simulink model "MPC_rpp"  (R2024a)
settings: Solver=FixedStepAuto  StartTime=0.0  StopTime=130  FixedStep=0.05  RelTol=1e-3
PostLoadFcn:
  | on_model_load
InitFcn:
  | on_model_start
StopFcn:
  | on_simulation_done
model workspace (MAT data in the model file):
  ActiveScenario.Id = "1e727098-795b-40af-9168-30502f01196e"
  ActiveScenario.Name = "Two steps"
  ActiveScenario.Description = ""
  ActiveScenario.ConstHorizonReference = 0
  ActiveScenario.ComponentType = "scenario"
  ActiveScenario.SimulationTime = 35
  ActiveScenario.Disturbance = struct()
  ActiveScenario.Subcomponents = "Disturbance"
  ActiveScenario.SystemIc = 0
  ActiveScenario.SystemParameterOverrides = struct()
  ActiveScenario.Reference = '/home/luka/fer/csbenchlab_gym/envs/marine_otter_velocity/data/references/1e727098-795b-40af-9168-30502f01196e_ref.mat'
  ActiveScenario.DisturbanceParameterOverrides = struct()
  ActiveScenario.NumEvaluations = 1
  ActiveScenario.RandomSeed = 42
  ActiveScenario.SystemParams.payload_mass = 5.1
  ActiveScenario.SystemParams.payload_location = [0; 0; 0]
  ActiveScenario.SystemParams.current_speed = 0
  ActiveScenario.SystemParams.current_direction = 0
  ActiveScenario.SystemParams.out_gain = 1
  GlobalReference = 0
  Scenarios(1).Id = "1e727098-795b-40af-9168-30502f01196e"
  Scenarios(1).Name = "Two steps"
  Scenarios(1).Description = ""
  Scenarios(1).ConstHorizonReference = 0
  Scenarios(1).ComponentType = "scenario"
  Scenarios(1).SimulationTime = 35
  Scenarios(1).Disturbance = struct()
  Scenarios(1).Subcomponents = "Disturbance"
  Scenarios(1).SystemIc = 0
  Scenarios(1).SystemParameterOverrides = struct()
  Scenarios(1).Reference = '/home/luka/fer/csbenchlab_gym/envs/marine_otter_velocity/data/references/1e727098-795b-40af-9168-30502f01196e_ref.mat'
  Scenarios(1).DisturbanceParameterOverrides = struct()
  Scenarios(1).NumEvaluations = 1
  Scenarios(1).RandomSeed = 42
  Scenarios(2).Id = "9caafca7-6b3d-4fd5-b43b-2d0badebda60"
  Scenarios(2).Name = "Five steps perturbed"
  Scenarios(2).Description = ""
  Scenarios(2).ConstHorizonReference = 0
  Scenarios(2).ComponentType = "scenario"
  Scenarios(2).SimulationTime = 35
  Scenarios(2).Disturbance.Id = '941af73e-12e7-42cf-853d-f79bb40068e7'
  Scenarios(2).Disturbance.Name = ''
  Scenarios(2).Disturbance.Description = ''
  Scenarios(2).Disturbance.LibVersionHash = ''
  Scenarios(2).Disturbance.Lib = 'csbenchlab'
  Scenarios(2).Disturbance.LibVersion = '0.0.1'
  Scenarios(2).Disturbance.PluginType = 'dist'
  Scenarios(2).Disturbance.PluginName = 'Gauss'
  Scenarios(2).Disturbance.PluginImplementation = 'mat'
  Scenarios(2).Disturbance.ParentComponentId = '9caafca7-6b3d-4fd5-b43b-2d0badebda60'
  Scenarios(2).Disturbance.ParentComponentType = 'scenario'
  Scenarios(2).Disturbance.ComponentType = 'disturbance'
  Scenarios(2).Disturbance.DestinationPath = 'disturbances'
  Scenarios(2).Subcomponents = "Disturbance"
  Scenarios(2).SystemIc = 0
  Scenarios(2).SystemParameterOverrides = struct()
  Scenarios(2).Reference = '/home/luka/fer/csbenchlab_gym/envs/marine_otter_velocity/data/references/9caafca7-6b3d-4fd5-b43b-2d0badebda60_ref.mat'
  Scenarios(2).DisturbanceParameterOverrides = struct()
  Scenarios(2).NumEvaluations = 1000
  Scenarios(2).RandomSeed = 42
  callbacks = dictionary
  callbacks.data.Version = 1
  callbacks.data.IsKeyCombined = 1
  callbacks.data.IsValueCombined = 1
  callbacks.data.Key = ["on_start:f41ef9e4-ba34-416c-84b6-7794956a3c04"; "on_start:b11ccfb6-c361-4845-af31-0c9bdb83000b"; "on_start:0f79c310-23a7-4b0d-9134-99211e5e6d76"; "on_start:68b44e77-22b1-45f7-8742-65551543004b"; "on_start:9c6c94ce-2741-455f-a8da-be6b073916ae"; "on_start:c9039aa6-3ac2-44ce-9131-deafcda314b8"; "on_load:4a0d1010-4549-4d51-b3a5-602e7c932b45"; "on_start:4a0d1010-4549-4d51-b3a5-602e7c932b45"; "on_end:4a0d1010-4549-4d51-b3a5-602e7c932b45"]
  callbacks.data.Value{1}.external_function__ = 1
  callbacks.data.Value{1}.function = 'configure_controller_params'
  callbacks.data.Value{1}.backend = 'm'
  callbacks.data.Value{1}.kwargs = struct()
  callbacks.data.Value{2}.external_function__ = 1
  callbacks.data.Value{2}.function = 'configure_controller_params'
  callbacks.data.Value{2}.backend = 'm'
  callbacks.data.Value{2}.kwargs = struct()
  callbacks.data.Value{3}.external_function__ = 1
  callbacks.data.Value{3}.function = 'configure_controller_params'
  callbacks.data.Value{3}.backend = 'm'
  callbacks.data.Value{3}.kwargs = struct()
  callbacks.data.Value{4}.external_function__ = 1
  callbacks.data.Value{4}.function = 'configure_controller_params'
  callbacks.data.Value{4}.backend = 'm'
  callbacks.data.Value{4}.kwargs = struct()
  callbacks.data.Value{5}.external_function__ = 1
  callbacks.data.Value{5}.function = 'configure_controller_params'
  callbacks.data.Value{5}.backend = 'm'
  callbacks.data.Value{5}.kwargs = struct()
  callbacks.data.Value{6}.external_function__ = 1
  callbacks.data.Value{6}.function = 'configure_controller_params'
  callbacks.data.Value{6}.backend = 'm'
  callbacks.data.Value{6}.kwargs = struct()
  callbacks.data.Value{7} = py.function
  callbacks.data.Value{8} = py.function
  callbacks.data.Value{9} = py.function
  env_name = 'MPC_rpp'
  extrinsic = 1
  gen_blocks.systems.systems.Name = 'CS System'
  gen_blocks.systems.systems.Handle = 'MPC_rpp/CS System'
  gen_blocks.systems.systems.Path = 'MPC_rpp/CS System'
  gen_blocks.systems.systems.Disturbance = []
  gen_blocks.systems.systems.Id = "4a0d1010-4549-4d51-b3a5-602e7c932b45"
  gen_blocks.systems.systems.Components.Name = 'Otter'
  gen_blocks.systems.systems.Components.Handle = 12585.0410156
  gen_blocks.systems.systems.Components.Path = 'MPC_rpp/CS System/Otter'
  gen_blocks.systems.systems.Components.Id = "4a0d1010-4549-4d51-b3a5-602e7c932b45"
  gen_blocks.systems.systems.Components.LibPath = "marine_lib_sys/Otter"
  gen_blocks.systems.systems.SignalSubsystem = []
  gen_blocks.systems.dims.Inputs = 1
  gen_blocks.systems.dims.Outputs = 1
  gen_blocks.controllers.Name = 'CS Controller1'
  gen_blocks.controllers.Handle = 'MPC_rpp/CS Controller1'
  gen_blocks.controllers.Path = 'MPC_rpp/CS Controller1'
  gen_blocks.controllers.Id = "81fc0e6f-2384-4969-ab33-4cc0b4a88dac"
  gen_blocks.controllers.Components.Name = 'MPC'
  gen_blocks.controllers.Components.Handle = 13345.0823975
  gen_blocks.controllers.Components.Path = 'MPC_rpp/CS Controller1/MPC'
  gen_blocks.controllers.Components.Id = "81fc0e6f-2384-4969-ab33-4cc0b4a88dac"
  gen_blocks.controllers.Components.LibPath = "csbenchlab_ctl/MPC"
  gen_blocks.controllers.Components.RefExtractor.Path = 'MPC_rpp/CS Controller1/ref_extractor_1'
  gen_blocks.controllers.IoHandles.inport_y.h = 12403.0534668
  gen_blocks.controllers.IoHandles.inport_y.p.Inport = []
  gen_blocks.controllers.IoHandles.inport_y.p.Outport = 12404.0565186
  gen_blocks.controllers.IoHandles.inport_y.p.Enable = []
  gen_blocks.controllers.IoHandles.inport_y.p.Trigger = []
  gen_blocks.controllers.IoHandles.inport_y.p.State = []
  gen_blocks.controllers.IoHandles.inport_y.p.LConn = []
  gen_blocks.controllers.IoHandles.inport_y.p.RConn = []
  gen_blocks.controllers.IoHandles.inport_y.p.Ifaction = []
  gen_blocks.controllers.IoHandles.inport_y.p.Reset = []
  gen_blocks.controllers.IoHandles.inport_y.p.Event = []
  gen_blocks.controllers.IoHandles.inport_yref.h = 12401.0418701
  gen_blocks.controllers.IoHandles.inport_yref.p.Inport = []
  gen_blocks.controllers.IoHandles.inport_yref.p.Outport = 12402.0541992
  gen_blocks.controllers.IoHandles.inport_yref.p.Enable = []
  gen_blocks.controllers.IoHandles.inport_yref.p.Trigger = []
  gen_blocks.controllers.IoHandles.inport_yref.p.State = []
  gen_blocks.controllers.IoHandles.inport_yref.p.LConn = []
  gen_blocks.controllers.IoHandles.inport_yref.p.RConn = []
  gen_blocks.controllers.IoHandles.inport_yref.p.Ifaction = []
  gen_blocks.controllers.IoHandles.inport_yref.p.Reset = []
  gen_blocks.controllers.IoHandles.inport_yref.p.Event = []
  gen_blocks.controllers.IoHandles.outport_u.h = 12405.0505371
  gen_blocks.controllers.IoHandles.outport_u.p.Inport = 12406.0664062
  gen_blocks.controllers.IoHandles.outport_u.p.Outport = []
  gen_blocks.controllers.IoHandles.outport_u.p.Enable = []
  gen_blocks.controllers.IoHandles.outport_u.p.Trigger = []
  gen_blocks.controllers.IoHandles.outport_u.p.State = []
  gen_blocks.controllers.IoHandles.outport_u.p.LConn = []
  gen_blocks.controllers.IoHandles.outport_u.p.RConn = []
  gen_blocks.controllers.IoHandles.outport_u.p.Ifaction = []
  gen_blocks.controllers.IoHandles.outport_u.p.Reset = []
  gen_blocks.controllers.IoHandles.outport_u.p.Event = []
  gen_blocks.controllers.IoHandles.outport_log.h = 12407.0563965
  gen_blocks.controllers.IoHandles.outport_log.p.Inport = 12408.0462646
  gen_blocks.controllers.IoHandles.outport_log.p.Outport = []
  gen_blocks.controllers.IoHandles.outport_log.p.Enable = []
  gen_blocks.controllers.IoHandles.outport_log.p.Trigger = []
  gen_blocks.controllers.IoHandles.outport_log.p.State = []
  gen_blocks.controllers.IoHandles.outport_log.p.LConn = []
  gen_blocks.controllers.IoHandles.outport_log.p.RConn = []
  gen_blocks.controllers.IoHandles.outport_log.p.Ifaction = []
  gen_blocks.controllers.IoHandles.outport_log.p.Reset = []
  gen_blocks.controllers.IoHandles.outport_log.p.Event = []
  gen_blocks.controllers.IoHandles.in_demux.p.Inport = 31230.0020752
  gen_blocks.controllers.IoHandles.in_demux.p.Outport = 31231.0020752
  gen_blocks.controllers.IoHandles.in_demux.p.Enable = []
  gen_blocks.controllers.IoHandles.in_demux.p.Trigger = []
  gen_blocks.controllers.IoHandles.in_demux.p.State = []
  gen_blocks.controllers.IoHandles.in_demux.p.LConn = []
  gen_blocks.controllers.IoHandles.in_demux.p.RConn = []
  gen_blocks.controllers.IoHandles.in_demux.p.Ifaction = []
  gen_blocks.controllers.IoHandles.in_demux.p.Reset = []
  gen_blocks.controllers.IoHandles.in_demux.p.Event = []
  gen_blocks.controllers.IoHandles.in_demux.h = 31229.0021973
  gen_blocks.controllers.IoHandles.in_demux_ref.p.Inport = 31226.0032959
  gen_blocks.controllers.IoHandles.in_demux_ref.p.Outport = 31227.0021973
  gen_blocks.controllers.IoHandles.in_demux_ref.p.Enable = []
  gen_blocks.controllers.IoHandles.in_demux_ref.p.Trigger = []
  gen_blocks.controllers.IoHandles.in_demux_ref.p.State = []
  gen_blocks.controllers.IoHandles.in_demux_ref.p.LConn = []
  gen_blocks.controllers.IoHandles.in_demux_ref.p.RConn = []
  gen_blocks.controllers.IoHandles.in_demux_ref.p.Ifaction = []
  gen_blocks.controllers.IoHandles.in_demux_ref.p.Reset = []
  gen_blocks.controllers.IoHandles.in_demux_ref.p.Event = []
  gen_blocks.controllers.IoHandles.in_demux_ref.h = 31225.0032959
  gen_blocks.controllers.IoHandles.out_mux.p.Inport = 13313.0822754
  gen_blocks.controllers.IoHandles.out_mux.p.Outport = 13315.0822754
  gen_blocks.controllers.IoHandles.out_mux.p.Enable = []
  gen_blocks.controllers.IoHandles.out_mux.p.Trigger = []
  gen_blocks.controllers.IoHandles.out_mux.p.State = []
  gen_blocks.controllers.IoHandles.out_mux.p.LConn = []
  gen_blocks.controllers.IoHandles.out_mux.p.RConn = []
  gen_blocks.controllers.IoHandles.out_mux.p.Ifaction = []
  gen_blocks.controllers.IoHandles.out_mux.p.Reset = []
  gen_blocks.controllers.IoHandles.out_mux.p.Event = []
  gen_blocks.controllers.IoHandles.out_mux.h = 13312.0822754
  gen_blocks.controllers.IoHandles.out_mux_log.p.Inport = 13317.0822754
  gen_blocks.controllers.IoHandles.out_mux_log.p.Outport = 13319.0822754
  gen_blocks.controllers.IoHandles.out_mux_log.p.Enable = []
  gen_blocks.controllers.IoHandles.out_mux_log.p.Trigger = []
  gen_blocks.controllers.IoHandles.out_mux_log.p.State = []
  gen_blocks.controllers.IoHandles.out_mux_log.p.LConn = []
  gen_blocks.controllers.IoHandles.out_mux_log.p.RConn = []
  gen_blocks.controllers.IoHandles.out_mux_log.p.Ifaction = []
  gen_blocks.controllers.IoHandles.out_mux_log.p.Reset = []
  gen_blocks.controllers.IoHandles.out_mux_log.p.Event = []
  gen_blocks.controllers.IoHandles.out_mux_log.h = 13316.0822754
  gen_blocks.controllers.IoHandles.ref_extractors.h = 13368.0825195
  gen_blocks.controllers.IoHandles.ref_extractors.name = 'ref_extractor_1'
  gen_blocks.controllers.IoHandles.ref_extractors.p.Inport = 13371.0822754
  gen_blocks.controllers.IoHandles.ref_extractors.p.Outport = 13416.0822754
  gen_blocks.controllers.IoHandles.ref_extractors.p.Enable = []
  gen_blocks.controllers.IoHandles.ref_extractors.p.Trigger = []
  gen_blocks.controllers.IoHandles.ref_extractors.p.State = []
  gen_blocks.controllers.IoHandles.ref_extractors.p.LConn = []
  gen_blocks.controllers.IoHandles.ref_extractors.p.RConn = []
  gen_blocks.controllers.IoHandles.ref_extractors.p.Ifaction = []
  gen_blocks.controllers.IoHandles.ref_extractors.p.Reset = []
  gen_blocks.controllers.IoHandles.ref_extractors.p.Event = []
  gen_blocks.controllers.IoHandles.adapters.in_mux.h = 13425.0823975
  gen_blocks.controllers.IoHandles.adapters.in_mux.p.Inport = 13426.0823975
  gen_blocks.controllers.IoHandles.adapters.in_mux.p.Outport = 13428.0822754
  gen_blocks.controllers.IoHandles.adapters.in_mux.p.Enable = []
  gen_blocks.controllers.IoHandles.adapters.in_mux.p.Trigger = []
  gen_blocks.controllers.IoHandles.adapters.in_mux.p.State = []
  gen_blocks.controllers.IoHandles.adapters.in_mux.p.LConn = []
  gen_blocks.controllers.IoHandles.adapters.in_mux.p.RConn = []
  gen_blocks.controllers.IoHandles.adapters.in_mux.p.Ifaction = []
  gen_blocks.controllers.IoHandles.adapters.in_mux.p.Reset = []
  gen_blocks.controllers.IoHandles.adapters.in_mux.p.Event = []
  gen_blocks.controllers.IoHandles.adapters.in_mux_ref.h = 13429.0822754
  gen_blocks.controllers.IoHandles.adapters.in_mux_ref.p.Inport = 13430.0822754
  gen_blocks.controllers.IoHandles.adapters.in_mux_ref.p.Outport = 13432.0822754
  gen_blocks.controllers.IoHandles.adapters.in_mux_ref.p.Enable = []
  gen_blocks.controllers.IoHandles.adapters.in_mux_ref.p.Trigger = []
  gen_blocks.controllers.IoHandles.adapters.in_mux_ref.p.State = []
  gen_blocks.controllers.IoHandles.adapters.in_mux_ref.p.LConn = []
  gen_blocks.controllers.IoHandles.adapters.in_mux_ref.p.RConn = []
  gen_blocks.controllers.IoHandles.adapters.in_mux_ref.p.Ifaction = []
  gen_blocks.controllers.IoHandles.adapters.in_mux_ref.p.Reset = []
  gen_blocks.controllers.IoHandles.adapters.in_mux_ref.p.Event = []
  gen_blocks.controllers.IoHandles.adapters.out_demux.h = 13433.0822754
  gen_blocks.controllers.IoHandles.adapters.out_demux.p.Inport = 13434.0822754
  gen_blocks.controllers.IoHandles.adapters.out_demux.p.Outport = 13435.0822754
  gen_blocks.controllers.IoHandles.adapters.out_demux.p.Enable = []
  gen_blocks.controllers.IoHandles.adapters.out_demux.p.Trigger = []
  gen_blocks.controllers.IoHandles.adapters.out_demux.p.State = []
  gen_blocks.controllers.IoHandles.adapters.out_demux.p.LConn = []
  gen_blocks.controllers.IoHandles.adapters.out_demux.p.RConn = []
  gen_blocks.controllers.IoHandles.adapters.out_demux.p.Ifaction = []
  gen_blocks.controllers.IoHandles.adapters.out_demux.p.Reset = []
  gen_blocks.controllers.IoHandles.adapters.out_demux.p.Event = []
  gen_blocks.controllers.IoHandles.adapters.scopes.y.h = 13437.0822754
  gen_blocks.controllers.IoHandles.adapters.scopes.y.p.Inport = [13438.0822754 13441.0822754]
  gen_blocks.controllers.IoHandles.adapters.scopes.y.p.Outport = []
  gen_blocks.controllers.IoHandles.adapters.scopes.y.p.Enable = []
  gen_blocks.controllers.IoHandles.adapters.scopes.y.p.Trigger = []
  gen_blocks.controllers.IoHandles.adapters.scopes.y.p.State = []
  gen_blocks.controllers.IoHandles.adapters.scopes.y.p.LConn = []
  gen_blocks.controllers.IoHandles.adapters.scopes.y.p.RConn = []
  gen_blocks.controllers.IoHandles.adapters.scopes.y.p.Ifaction = []
  gen_blocks.controllers.IoHandles.adapters.scopes.y.p.Reset = []
  gen_blocks.controllers.IoHandles.adapters.scopes.y.p.Event = []
  gen_blocks.controllers.IoHandles.adapters.scopes.u.h = 13439.0822754
  gen_blocks.controllers.IoHandles.adapters.scopes.u.p.Inport = 13440.0822754
  gen_blocks.controllers.IoHandles.adapters.scopes.u.p.Outport = []
  gen_blocks.controllers.IoHandles.adapters.scopes.u.p.Enable = []
  gen_blocks.controllers.IoHandles.adapters.scopes.u.p.Trigger = []
  gen_blocks.controllers.IoHandles.adapters.scopes.u.p.State = []
  gen_blocks.controllers.IoHandles.adapters.scopes.u.p.LConn = []
  gen_blocks.controllers.IoHandles.adapters.scopes.u.p.RConn = []
  gen_blocks.controllers.IoHandles.adapters.scopes.u.p.Ifaction = []
  gen_blocks.controllers.IoHandles.adapters.scopes.u.p.Reset = []
  gen_blocks.controllers.IoHandles.adapters.scopes.u.p.Event = []
  gen_blocks.controllers.IoHandles.adapters.cont.h = 13345.0823975
  gen_blocks.controllers.IoHandles.adapters.cont.p.Inport = [13348.0823975 13349.0823975 13350.0823975]
  gen_blocks.controllers.IoHandles.adapters.cont.p.Outport = [13361.0822754 13362.0822754]
  gen_blocks.controllers.IoHandles.adapters.cont.p.Enable = []
  gen_blocks.controllers.IoHandles.adapters.cont.p.Trigger = []
  gen_blocks.controllers.IoHandles.adapters.cont.p.State = []
  gen_blocks.controllers.IoHandles.adapters.cont.p.LConn = []
  gen_blocks.controllers.IoHandles.adapters.cont.p.RConn = []
  gen_blocks.controllers.IoHandles.adapters.cont.p.Ifaction = []
  gen_blocks.controllers.IoHandles.adapters.cont.p.Reset = []
  gen_blocks.controllers.IoHandles.adapters.cont.p.Event = []
  gen_blocks.controllers.IoHandles.adapters.Mux.Inputs = 1
  gen_blocks.controllers.IoHandles.adapters.Mux.Outputs = 1
  gen_blocks.controllers.Estimator = []
  gen_blocks.controllers.Disturbance = []
  gen_blocks.controllers.SignalSubsystem = []
  gen_blocks.cs_blocks = {'MPC_rpp/CS Controller1'; 'MPC_rpp/CS Controller1/MPC'; 'MPC_rpp/CS System'; 'MPC_rpp/CS System/Otter'}
  gen_data_dictionary = Simulink.data.Dictionary
  id_to_params_path_map = dictionary
  id_to_params_path_map.data.Version = 1
  id_to_params_path_map.data.IsKeyCombined = 1
  id_to_params_path_map.data.IsValueCombined = 1
  id_to_params_path_map.data.Key = ["4a0d1010-4549-4d51-b3a5-602e7c932b45"; "81fc0e6f-2384-4969-ab33-4cc0b4a88dac"; "941af73e-12e7-42cf-853d-f79bb40068e7"]
  id_to_params_path_map.data.Value = ["MPC_rpp_params.sys.Otter"; "MPC_rpp_params.ctl.MPC"; "MPC_rpp_params.Subcomponents.FiveStepsPerturbed.x"]
  model_info.Metadata.Id = "e28b07d8-94b6-4791-bb8b-7f4e501fe7eb"
  model_info.Metadata.Name = "marine_otter_velocity"
  model_info.Metadata.Ts = 0.05
  model_info.Metadata.ComponentType = "metadata"
  model_info.Metadata.CoderExtrinsic = 1
  model_info.Metadata.Metadata.Authors = "Luka Mandic"
  model_info.Metadata.Metadata.Version = "0.1"
  model_info.Metadata.Metadata.License = "Apache v2"
  model_info.Metadata.Metadata.Tags = "marine,velocity"
  model_info.Metadata.Metadata.Created = ""
  model_info.Metadata.Metadata.Modified = ""
  model_info.Controllers.Id = "81fc0e6f-2384-4969-ab33-4cc0b4a88dac"
  model_info.Controllers.Name = "MPC"
  model_info.Controllers.Description = ""
  model_info.Controllers.LibVersionHash = ""
  model_info.Controllers.Lib = "csbenchlab"
  model_info.Controllers.LibVersion = "0.0.1"
  model_info.Controllers.PluginType = "ctl"
  model_info.Controllers.PluginName = "MPC"
  model_info.Controllers.IsComposable = 0
  model_info.Controllers.RefHorizon = 1
  model_info.Controllers.Mux.Inputs = 1
  model_info.Controllers.Mux.Outputs = 1
  model_info.Controllers.Subcomponents = "Subcontrollers"
  model_info.Controllers.Disturbance = struct()
  model_info.Controllers.ComponentType = "controller"
  model_info.Controllers.PluginImplementation = "slx"
  model_info.Controllers.Subcontrollers = []
  model_info.System.Id = "4a0d1010-4549-4d51-b3a5-602e7c932b45"
  model_info.System.Name = "Otter"
  model_info.System.Description = ""
  model_info.System.LibVersionHash = ""
  model_info.System.Lib = "marine_lib"
  model_info.System.LibVersion = "0.0.1"
  model_info.System.PluginType = "sys"
  model_info.System.PluginName = "Otter"
  model_info.System.Subcomponents = "Disturbance"
  model_info.System.Disturbance = struct()
  model_info.System.ComponentType = "system"
  model_info.System.PluginImplementation = "slx"
  model_info.Metrics.Id = "9c8fc09b-5b47-4f25-8326-e915b50c92f8"
  model_info.Metrics.Name = "Plot out wit reference"
  model_info.Metrics.Description = ""
  model_info.Metrics.ComponentType = "metric"
  model_info.Scenarios(1).Id = "1e727098-795b-40af-9168-30502f01196e"
  model_info.Scenarios(1).Name = "Two steps"
  model_info.Scenarios(1).Description = ""
  model_info.Scenarios(1).ConstHorizonReference = 0
  model_info.Scenarios(1).ComponentType = "scenario"
  model_info.Scenarios(1).SimulationTime = 35
  model_info.Scenarios(1).Disturbance = struct()
  model_info.Scenarios(1).Subcomponents = "Disturbance"
  model_info.Scenarios(2).Id = "9caafca7-6b3d-4fd5-b43b-2d0badebda60"
  model_info.Scenarios(2).Name = "Five steps perturbed"
  model_info.Scenarios(2).Description = ""
  model_info.Scenarios(2).ConstHorizonReference = 0
  model_info.Scenarios(2).ComponentType = "scenario"
  model_info.Scenarios(2).SimulationTime = 35
  model_info.Scenarios(2).Disturbance.Id = "941af73e-12e7-42cf-853d-f79bb40068e7"
  model_info.Scenarios(2).Disturbance.Name = ""
  model_info.Scenarios(2).Disturbance.Description = ""
  model_info.Scenarios(2).Disturbance.LibVersionHash = ""
  model_info.Scenarios(2).Disturbance.Lib = "csbenchlab"
  model_info.Scenarios(2).Disturbance.LibVersion = "0.0.1"
  model_info.Scenarios(2).Disturbance.PluginType = "dist"
  model_info.Scenarios(2).Disturbance.PluginName = "Gauss"
  model_info.Scenarios(2).Disturbance.PluginImplementation = "mat"
  model_info.Scenarios(2).Disturbance.ParentComponentId = "9caafca7-6b3d-4fd5-b43b-2d0badebda60"
  model_info.Scenarios(2).Disturbance.ParentComponentType = "scenario"
  model_info.Scenarios(2).Disturbance.ComponentType = "disturbance"
  model_info.Scenarios(2).Disturbance.DestinationPath = "disturbances"
  model_info.Scenarios(2).Disturbance.ParentComponentName = "Five steps perturbed"
  model_info.Scenarios(2).Subcomponents = "Disturbance"
  model_info.IsControlEnvironment = 0
  model_type = 'scenario'
  old_params.Subcomponents.FiveStepsPerturbed.x.mu = 0
  old_params.Subcomponents.FiveStepsPerturbed.x.sigma = 0.05
  old_params.sys.Otter.payload_mass = 5.1
  old_params.sys.Otter.payload_location = [0; 0; 0]
  old_params.sys.Otter.current_speed = 0
  old_params.sys.Otter.current_direction = 0
  old_params.sys.Otter.out_gain = 1
  old_params.ctl.MPC.mpc_path = [100 97 116 97 47 109 112 99 46 109 97 116]
  old_params.ComponentContext = dictionary
  old_params.ComponentContext.data.Version = 1
  old_params.ComponentContext.data.IsKeyCombined = 1
  old_params.ComponentContext.data.IsValueCombined = 1
  old_params.ComponentContext.data.Key = ["4a0d1010-4549-4d51-b3a5-602e7c932b45"; "81fc0e6f-2384-4969-ab33-4cc0b4a88dac"; "941af73e-12e7-42cf-853d-f79bb40068e7"]
  old_params.ComponentContext.data.Value = ["/home/luka/fer/csbenchlab_gym/envs/marine_otter_velocity/parts/systems/4a0d1010-4549-4d51-b3a5-602e7c932b45"; "/home/luka/fer/csbenchlab_gym/envs/marine_otter_velocity/parts/controllers/81fc0e6f-2384-4969-ab33-4cc0b4a88dac"; "/home/luka/fer/csbenchlab_gym/envs/marine_otter_velocity/parts/scenarios/9caafca7-6b3d-4fd5-b43b-2d0badebda60/subcomponents/disturbances/941af73e-12e7-42cf-853d-f79bb40068e7"]
  old_params.EnvPath = '/home/luka/fer/csbenchlab_gym/envs/marine_otter_velocity'
undefined symbols (not defined in the file): rpp_params
libraries: csbenchlab_ctl x1, marine_lib_sys x1, slpidlib x1, cmmi_lib x1
PostSaveFcn:
  | on_model_save
settings Model: DataDictionary=MPC_rpp_bus_types.sldd  Creator=luka  LastModifiedBy=luka

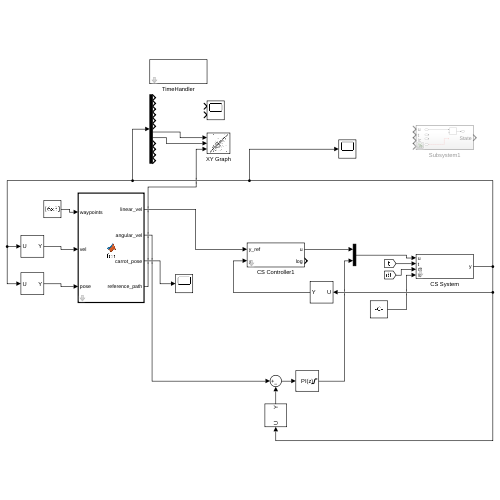
[thumbnail: Simulink's stored preview of the top-level diagram]
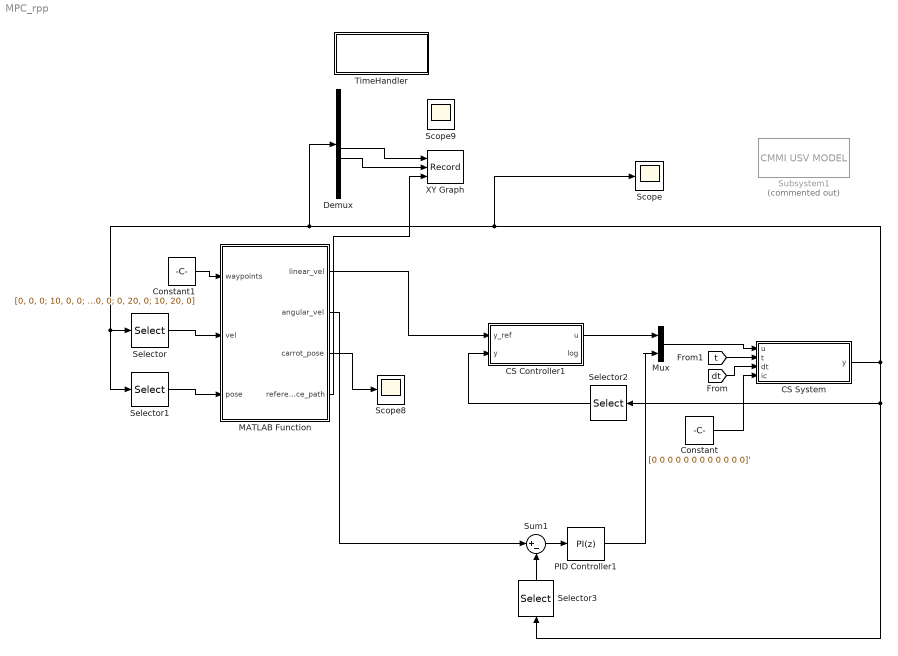
== system MPC_rpp ==
  CS Controller1 : Subsystem  Tag=__cs_template;__cs_comptype:ctl
      mask DialogControl ParameterGroupVar Prompt: Params
  CS System : Subsystem  Tag=__cs_template;__cs_comptype:sys
      mask DialogControl ParameterGroupVar Prompt: Params
  Constant : Constant  Value=[0 0 0 0 0 0 0 0 0 0 0 0]'
  Constant1 : Constant  Value=[0, 0, 0; 10, 0, 0; 10 10, 0; 0, 10, 0; 0, 20, 0; 10, 20, 0]
  Demux : Demux  Outputs=12
  MATLAB Function : MATLAB Function  TreatAsAtomicUnit=on  mask{params=rpp_params}
  Mux : Mux  Inputs=2
  PID Controller1 : slpidlib/PID Controller  Controller=PI  Form=Parallel  TimeDomain=Discrete-time  UseExternalTs=off  SampleTime=0.05  IntegratorMethod=Forward Euler  FilterMethod=Forward Euler  ControllerParametersSource=internal  P=500  I=400  UseKiTs=off  D=0.0826067692513504  UseExternalDerivativeSource=off  N=21.0121039234625  UseFilter=on  TunerSelectOption=Transfer Function Based (PID Tuner App)  InitialConditionSource=internal  InitialConditionForIntegrator=0  InitialConditionForFilter=0  DifferentiatorICPrevScaledInput=0  ExternalReset=none  TrackingMode=off  Kt=1  LimitOutput=on  SatLimitsSource=internal  UpperSaturationLimit=300  LowerSaturationLimit=-150  LinearizeAsGain=on  AntiWindupMode=clamping  Kb=1  LimitIntegrator=on  UpperIntegratorSaturationLimit=300  LowerIntegratorSaturationLimit=-150  POutMin=[]  POutMax=[]  IOutMin=[]  IOutMax=[]  DOutMin=[]  DOutMax=[]  NOutMin=[]  NOutMax=[]  SumOutMin=[]  SumOutMax=[]  SaturationOutMin=[]  SaturationOutMax=[]  PParamMin=[]  PParamMax=[]  IParamMin=[]  IParamMax=[]  DParamMin=[]  DParamMax=[]  NParamMin=[]  NParamMax=[]  KbParamMin=[]  KbParamMax=[]  KtParamMin=[]  KtParamMax=[]  KbOutMin=[]  KbOutMax=[]  KtOutMin=[]  KtOutMax=[]  IntegratorOutMin=[]  IntegratorOutMax=[]  FilterOutMin=[]  FilterOutMax=[]  SumI1OutMin=[]  SumI1OutMax=[]  SumI2OutMin=[]  SumI2OutMax=[]  SumI3OutMin=[]  SumI3OutMax=[]  SumI4OutMin=[]  SumI4OutMax=[]  SumDOutMin=[]  SumDOutMax=[]  DifferentiatorOutMin=[]  DifferentiatorOutMax=[]  FilterDiffOutCoefMin=[]  FilterDiffOutCoefMax=[]  ReciprocalOutMin=[]  ReciprocalOutMax=[]  SumDenOutMin=[]  SumDenOutMax=[]  SumNumOutMin=[]  SumNumOutMax=[]  DivideOutMin=[]  DivideOutMax=[]  UdiffTsProdOutMin=[]  UdiffTsProdOutMax=[]  NTsProdOutMin=[]  NTsProdOutMax=[]  UintegralTsProdOutMin=[]  UintegralTsProdOutMax=[]  UngainTsProdOutMin=[]  UngainTsProdOutMax=[]  ClampingZeroOutDataTypeStr=Inherit: Inherit via back propagation  ClampingZeroOutMin=[]  ClampingZeroOutMax=[]  FilterDenConstantOutDataTypeStr=Inherit: Inherit via back propagation  FilterDenConstantOutMin=[]  FilterDenConstantOutMax=[]  PCopyOutDataTypeStr=Inherit: Inherit via back propagation  PCopyOutMin=[]  PCopyOutMax=[]  NCopyOutDataTypeStr=Inherit: Inherit via back propagation  NCopyOutMin=[]  NCopyOutMax=[]  IntegratorContinuousStateAttributes=''  IntegratorStateMustResolveToSignalObject=off  IntegratorRTWStateStorageClass=Auto  FilterContinuousStateAttributes=''  FilterStateMustResolveToSignalObject=off  FilterRTWStateStorageClass=Auto  ParallelPVariant=InternalParameters  IdealPVariant=Disabled  IVariant=InternalParameters  DVariant=Disabled  IntegratorVariant=Discrete  SatVariant=Enabled  AWVariant=DiscClampingParallel  PCopyVariant=Disabled  TRVariant=Disabled  FdbkBlocksVariant=Forward  IdealPFdbkVariant=Disabled  SatFdbkVariant=Disabled  DerivativeFilterVariant=Disabled  NVariant=Disabled  NCopyVariant=Disabled_SignalSpec  FilterICVariant=Disabled  IntegratorICVariant=InternalICs  ExternalResetVariant=Disabled  TRSumVariant=Passthrough  SumFdbkVariant=Disabled  SumVariant=Sum_PI  TsampFilterVariant=InternalTs  TsampNgainVariant=Passthrough  TsampIntegralVariant=Disabled_SignalSpec  ExternalSaturationOutDataTypeStr=Inherit: Same as second input  DerivativeSourceVariant=Disabled
  Scope : Scope
  Scope8 : Scope
  Scope9 : Scope  NumInputPorts=2
  Selector : Selector  InputPortWidth=12  IndexOptions=Index vector (dialog)  Indices=[1 2 6]  OutputSizes=1
  Selector1 : Selector  InputPortWidth=12  IndexOptions=Index vector (dialog)  Indices=[7 8 12]  OutputSizes=1
  Selector2 : Selector  InputPortWidth=12  IndexOptions=Index vector (dialog)  Indices=[1]  OutputSizes=1
  Selector3 : Selector  InputPortWidth=12  IndexOptions=Index vector (dialog)  Indices=[6]  OutputSizes=1
  Subsystem1 : cmmi_lib/CMMI USV MODEL  Commented=on  SystemSampleTime=-1  VariantActivationTime=update diagram  AllowFlexibleInterface=on  Latency=0  AutoFrameSizeCalculation=off
      link override Subsystem/Saturation: UpperLimit=1  LowerLimit=-1
  Sum1 : Sum  Inputs=|+-
  TimeHandler : Subsystem
      mask DialogControl ParameterGroupVar Prompt: Params
  XY Graph : Record  FileSettingsInternal="{\"entries\":[{\"content\":{\"excelSettings\":{\"content\":{},\"type\":\"Streamout.ExcelSettings\"}},\"type\":\"Streamout.FileSettingStorage\",\"uuid\":\"\"}],\"packageUris\":[\"http:\\/\\/schema.mathworks.com\\/mf0\\/streamout_blocks\\/R2020a\"],\"version\":\"1.0\"}"  Layout=[1 1]  SignalsInternal="{\"entries\":[{\"content\":{\"signals\":[{\"content\":{\"blockPath\":[],\"dimensions\":[1],\"domain\":\"\",\"lineColor\":\"#139fff\",\"lineWidth\":2,\"port\":1,\"sid\":[\"\"],\"signalID\":1,\"signalName\":\"Demux:7\"},\"type\":\"RecordBlkView.Signal\",\"uuid\":\"\"},{\"content\":{\"blockPath\":[],\"dimensions\":[1],\"domain\":\"\",\"lineColor\":\"#ff6929\",\"lineWidth\":2,\"port\":2,\"sid\":[\"\"],\"signalID\":2,\"signalName\":\"Demux:8\"},\"type\":\"RecordBlkView.Signal\",\"uuid\":\"\"},{\"content\":{\"blockPath\":[],\"dimensions\":[501,3],\"domain\":\"\",\"hasChildren\":true,\"lineColor\":\"#b746ff\",\"lineWidth\":2,\"port\":3,\"sid\":[\"\"],\"signalID\":3,\"signalName\":\"MATLAB Function:4\"},\"type\":\"RecordBlkView.Signal\",\"uuid\":\"\"},{\"content\":{\"blockPath\":[],\"channel\":[1,1],\"dimensions\":[501,3],\"domain\":\"\",\"lineColor\":\"#64d413\",\"lineWidth\":2,\"parentID\":3,\"port\":3,\"sid\":[\"\"],\"signalID\":4,\"signalName\":\"MATLAB Function:4\"},\"type\":\"RecordBlkView.Signal\",\"uuid\":\"\"}]},\"type\":\"RecordBlkView.InputSignals\",\"uuid\":\"\"}],\"packageUris\":[\"http:\\/\\/schema.mathworks.com\\/mf0\\/streamout_blocks\\/R2020a\"],\"version\":\"1.0\"}"  VisualizationBindings="{\"xyplotplugin\":{\"info\":[{\"series\":[],\"subplotID\":1}]}}"  CompatibilityTag=XY
  wires:
  Constant1/1 -> MATLAB Function/1(waypoints)
  Selector/1 -> MATLAB Function/2(vel)
  Selector1/1 -> MATLAB Function/3(pose)
  MATLAB Function/3(carrot_pose) -> Scope8/1
  CS Controller1/1(u) -> Mux/1
  Mux/1 -> CS System/1(u)
  MATLAB Function/1(linear_vel) -> CS Controller1/1(y_ref)
  [dt] -> CS System/3(dt)
  [t] -> CS System/2(t)
  Constant/1 -> CS System/4(ic)
  Selector2/1 -> CS Controller1/2(y)
  Sum1/1 -> PID Controller1/1
  CS System/1(y) -> Selector2/1, Selector3/1, Scope/1, Selector1/1, Selector/1, Demux/1
  Selector3/1 -> Sum1/2
  MATLAB Function/2(angular_vel) -> Sum1/1
  PID Controller1/1 -> Mux/2
  MATLAB Function/4(reference_path) -> XY Graph/3
  Demux/7 -> XY Graph/1
  Demux/8 -> XY Graph/2

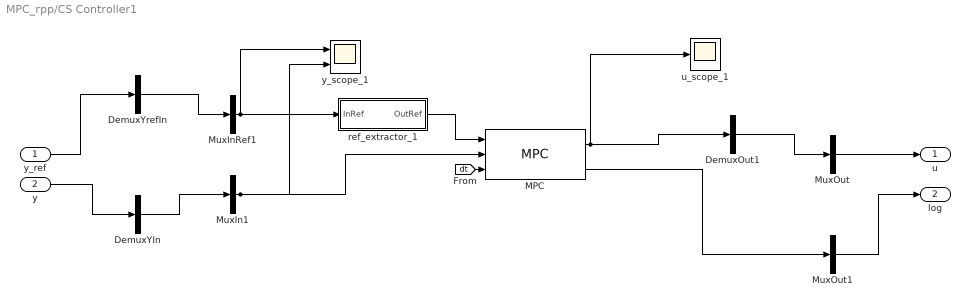
== system MPC_rpp/CS Controller1 ==
  y_ref : Inport  PortDimensions=1
  y : Inport  Port=2  PortDimensions=1
  DemuxOut1 : Demux  Outputs=1
  DemuxYIn : Demux  Outputs=1
  DemuxYrefIn : Demux  Outputs=1
  MPC : csbenchlab_ctl/MPC  Tag=__cs_slx_ctl;__cs_comptype:ctl;__cs_compimpl:slx;  mpc_path=MPC_rpp_params.ctl.MPC.mpc_path  iid__=[56 49 102 99 48 101 54 102 45 50 51 56 52 45 52 57 54 57 45 97 98 51 51 45 52 99 99 48 98 52 97 56 56 100 97 99]  pid__=[77 80 67 58 99 115 98 101 110 99 104 108 97 98]  params=MPC_rpp_params.ctl.MPC  params_struct_name=MPC_rpp_params.ctl.MPC
  MuxIn1 : Mux  Inputs=1
  MuxInRef1 : Mux  Inputs=1
  MuxOut : Mux  Inputs=1
  MuxOut1 : BusCreator  Inputs=1
  ref_extractor_1 : Subsystem
  u_scope_1 : Scope
  y_scope_1 : Scope  NumInputPorts=2
  u : Outport  PortDimensions=1
  log : Outport  Port=2
  wires:
  [dt] -> MPC/3
  y/1 -> DemuxYIn/1
  y_ref/1 -> DemuxYrefIn/1
  MuxOut/1 -> u/1
  MuxOut1/1 -> log/1
  MuxInRef1/1 -> ref_extractor_1/1(InRef), y_scope_1/1
  ref_extractor_1/1(OutRef) -> MPC/1
  MuxIn1/1 -> MPC/2, y_scope_1/2
  MPC/1 -> DemuxOut1/1, u_scope_1/1
  MPC/2 -> MuxOut1/1
  DemuxYIn/1 -> MuxIn1/1
  DemuxYrefIn/1 -> MuxInRef1/1
  DemuxOut1/1 -> MuxOut/1

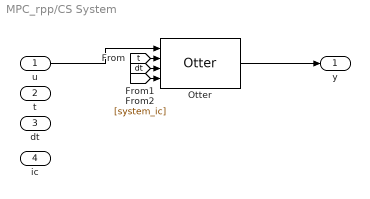
== system MPC_rpp/CS System ==
  u : Inport
  t : Inport  Port=2
  dt : Inport  Port=3
  ic : Inport  Port=4
  Otter : marine_lib_sys/Otter  Tag=system;__cs_slx_sys;__cs_comptype:sys;__cs_compimpl:slx;  payload_mass=MPC_rpp_params.sys.Otter.payload_mass  payload_location=MPC_rpp_params.sys.Otter.payload_location  current_speed=MPC_rpp_params.sys.Otter.current_speed  current_direction=MPC_rpp_params.sys.Otter.current_direction  out_gain=MPC_rpp_params.sys.Otter.out_gain  iid__=[52 97 48 100 49 48 49 48 45 52 53 52 57 45 52 100 53 49 45 98 51 97 53 45 54 48 50 101 55 99 57 51 50 98 52 53]  pid__=[79 116 116 101 114 58 109 97 114 105 110 101 95 108 105 98]  params=ActiveScenario.SystemParams  params_struct_name=MPC_rpp_params.sys.Otter
  y : Outport
  wires:
  u/1 -> Otter/1
  Otter/1 -> y/1
  [t] -> Otter/2
  [dt] -> Otter/3
  [system_ic] -> Otter/4

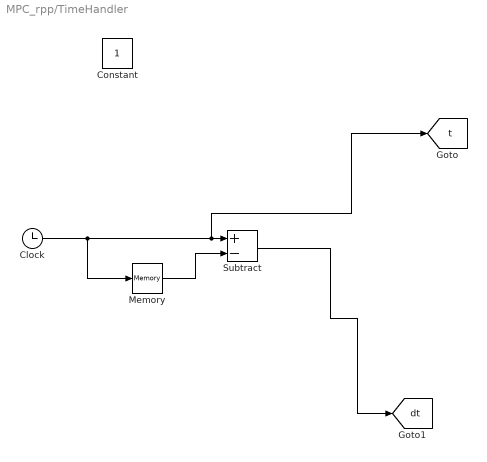
== system MPC_rpp/TimeHandler ==
  Clock : Clock
  Constant : Constant
  Memory : Memory
  Subtract : Sum  Inputs=+-
  tag scope: dt=global, t=global
  wires:
  Clock/1 -> [t], Subtract/1, Memory/1
  Memory/1 -> Subtract/2
  Subtract/1 -> [dt]

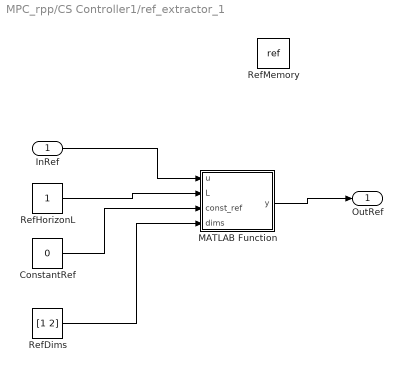
== system MPC_rpp/CS Controller1/ref_extractor_1 ==
  InRef : Inport
  ConstantRef : Constant  Value=0
  MATLAB Function : MATLAB Function  TreatAsAtomicUnit=on
  RefDims : Constant  Value=[1 2]
  RefHorizonL : Constant
  RefMemory : DataStoreMemory  DataStoreName=ref  WriteAfterWriteMsg=warning  ShowAdditionalParam=off  OutDataTypeStr=double
  OutRef : Outport
  wires:
  ConstantRef/1 -> MATLAB Function/3(const_ref)
  RefDims/1 -> MATLAB Function/4(dims)
  RefHorizonL/1 -> MATLAB Function/2(L)
  InRef/1 -> MATLAB Function/1(u)
  MATLAB Function/1(y) -> OutRef/1

== matlab function MPC_rpp/MATLAB Function ==
  settings: updateMethod=DISCRETE
  data: waypoints input; vel input; pose input; linear_vel output; params parameter; angular_vel output; carrot_pose output size=[1 3]; reference_path output
function [linear_vel, angular_vel, carrot_pose, reference_path] = fcn(waypoints, vel, pose, params)

    persistent global_path idx initial_global_path
    use_waypoints = 1;
    num_divs = 100;        
    if isempty(global_path)

        if use_waypoints
            global_path = zeros((height(waypoints)-1) * num_divs+1, 3);
            global_path(1, :) = waypoints(1, :);
            for i=1:length(waypoints)-1
                global_path(2 + (i-1)*num_divs : i*num_divs+1, :) = get_traj_between(waypoints(i, :), waypoints(i+1, :), num_divs);
            end
            idx = 1;
        else
            global_path = zeros((height(waypoints)-1) * num_divs+1, 3);
            global_path(1, :) = waypoints(1, :);
            k=5;
            kx=1.3;
            ky=0;
            L = 200;
            N = 5;
            theta=linspace(0, 2*N*pi, L);
            r = k*theta;
            x = k*(cos(theta)-1) + kx*theta;
            y = k*sin(theta) + ky*theta;
            global_path(2:L+1, :) = [x' y' zeros(L, 1)] + repmat(global_path(1, :), L, 1);
            global_path(L+2:end, :) = repmat(global_path(L+1, :), length(global_path) - L-1, 1);
            idx = 1;
        end
        initial_global_path = global_path;
    end
    reference_path = initial_global_path;
    coder.extrinsic('regulated_pure_pursuit')
    coder.extrinsic('transform_path_to_local')
    coder.extrinsic('prune_global_path')
    linear_vel = 0; angular_vel = 0;
    carrot_pose = [0,0,0];
    idx = prune_global_path(pose, global_path, idx, 0.8 * params.lookahead_dist, 2);
    local_path = transform_path_to_local(pose, global_path(idx:end, :));
    [linear_vel, angular_vel, carrot] = regulated_pure_pursuit(local_path, vel, params);
    carrot_pose(1:2) = carrot;
end

== matlab function MPC_rpp/CS Controller1/ref_extractor_1/MATLAB Function ==
  settings: updateMethod=DISCRETE
  data: u input; L input; const_ref input; dims input; y output; ref data_store_memory; GlobalReference parameter
function y = fcn(u, L, const_ref, dims, GlobalReference)

persistent cnt
global ref

if isempty(cnt)
    cnt = 0;
end

if GlobalReference == 0
    y = repmat(u, 1);
    return;
end


cnt = cnt+1;

horizon_end = cnt+L-1;
if L > 1 
   if horizon_end > length(GlobalReference)
        if size(ref, 1) == size(u, 1)
            y = permute(ref, [2, 1]);
        else
            y = ref;
        end       
        return
   end

   if size(ref, 1) == size(u, 1)
      
      if const_ref == 0
        ref(:, :) = GlobalReference(cnt:horizon_end, dims)';
      else
        ref(:, :) = repmat(GlobalReference(cnt, dims)', 1, L);
      end
      y = permute(ref, [2, 1]);
   else
      if const_ref == 0
        ref(1:L, :) = GlobalReference(cnt:horizon_end, dims);
      else
        ref(1:L, :) = repmat(GlobalReference(cnt, dims), L, 1);
      end
      y = ref;
   end
else
   if size(ref, 1) == size(u, 1)
       ref = u;
       y = permute(ref, [2, 1]);
   else
      ref(1, :) = u';
      y = ref;
   end
end
